simulink model "power_sys_sim"  (R2023b)
settings: Solver=VariableStepAuto  StartTime=0.0  StopTime=0.1  FixedStep=0.00001  RelTol=1e-3
libraries: spsThyristorLib x5, spsVoltageMeasurementLib x5, spsCurrentMeasurementLib x4, spsDiodeLib x4, spsSeriesRLCBranchLib x4, spsACVoltageSourceLib x3, spsMeanLib x2, sps_lib x1
settings Model: Creator=yuanluochen  LastModifiedBy=yuanluochen

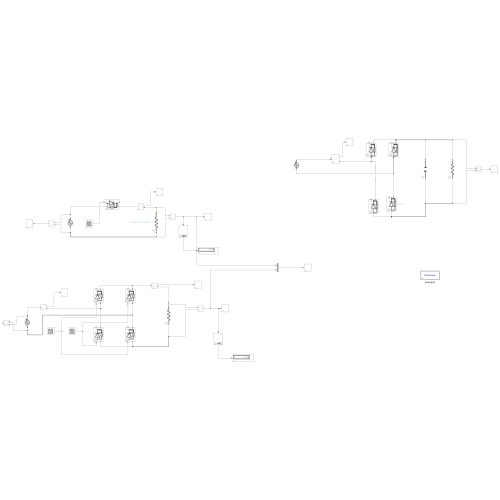
[thumbnail: Simulink's stored preview of the top-level diagram]
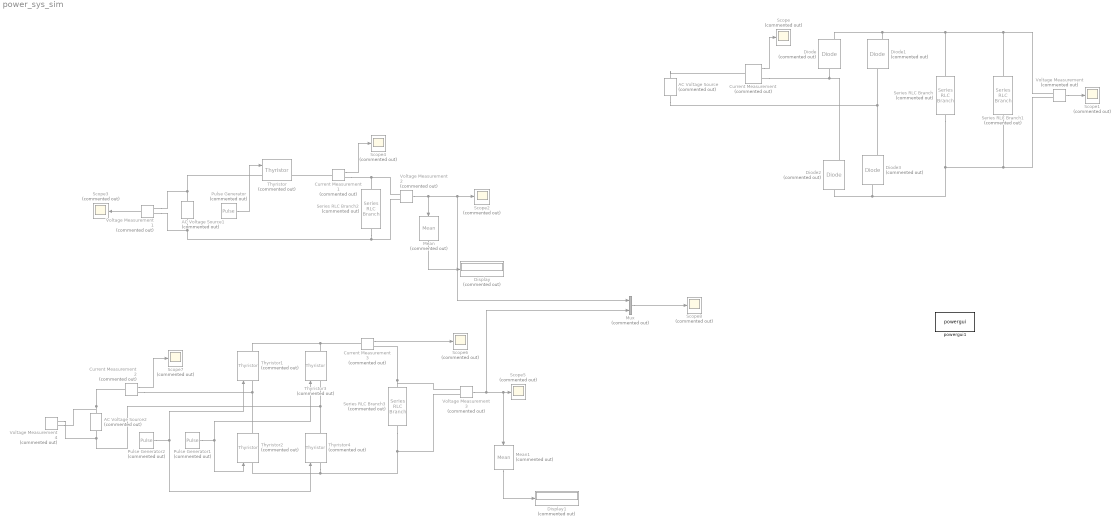
== system power_sys_sim ==
  AC Voltage Source : spsACVoltageSourceLib/AC Voltage Source  Commented=on  Amplitude=220*sqrt(2)  Phase=0  Frequency=50  SampleTime=0  Measurements=None  BusType=swing  Pref=10e3  Qref=0  Qmin=-inf  Qmax=+inf
  AC Voltage Source1 : spsACVoltageSourceLib/AC Voltage Source  Commented=on  Amplitude=220*sqrt(2)  Phase=0  Frequency=50  SampleTime=0  Measurements=None  BusType=swing  Pref=10e3  Qref=0  Qmin=-inf  Qmax=+inf
  AC Voltage Source2 : spsACVoltageSourceLib/AC Voltage Source  Commented=on  Amplitude=220*sqrt(2)  Phase=0  Frequency=50  SampleTime=0  Measurements=None  BusType=swing  Pref=10e3  Qref=0  Qmin=-inf  Qmax=+inf
  Current Measurement{,1..3} (4 alike) : spsCurrentMeasurementLib/Current Measurement  Commented=on  PhasorSimulation=off  OutputType=Complex  PSBequivalent=0
  Diode{,1..3} (4 alike) : spsDiodeLib/Diode  Commented=on  Ron=0.001  Lon=0  Vf=0.8  IC=0  UseSnubber=0  Rs=500  Cs=250e-9  Measurements=on
  Display : Display  Commented=on
  Display1 : Display  Commented=on
  Mean : spsMeanLib/Mean  Commented=on  Freq=50  Vinit=0  Ts=0
  Mean1 : spsMeanLib/Mean  Commented=on  Freq=50  Vinit=0  Ts=0
  Mux : Mux  Commented=on  Inputs=2
  Pulse Generator : DiscretePulseGenerator  Commented=on  PulseType=Time based  Amplitude=3  Period=0.02  PulseWidth=10  PhaseDelay=60/360*0.02
  Pulse Generator1 : DiscretePulseGenerator  Commented=on  PulseType=Time based  Amplitude=3  Period=0.02  PulseWidth=10  PhaseDelay=60/360*0.02+0.01
  Pulse Generator2 : DiscretePulseGenerator  Commented=on  PulseType=Time based  Amplitude=3  Period=0.02  PulseWidth=10  PhaseDelay=60/360*0.02
  Scope{,1..8} (9 alike) : Scope  Commented=on
  Series RLC Branch : spsSeriesRLCBranchLib/Series RLC Branch  Commented=on  LConnTagsString=__new0  RConnTagsString=__new0  BranchType=C  Resistance=1  Inductance=1e-3  SetiL0=off  InitialCurrent=0  Capacitance=0.001  Setx0=off  InitialVoltage=0  Measurements=None
  Series RLC Branch1 : spsSeriesRLCBranchLib/Series RLC Branch  Commented=on  LConnTagsString=__new0  RConnTagsString=__new0  BranchType=R  Resistance=20  Inductance=1e-3  SetiL0=off  InitialCurrent=0  Capacitance=1e-6  Setx0=off  InitialVoltage=0  Measurements=None
  Series RLC Branch2 : spsSeriesRLCBranchLib/Series RLC Branch  Commented=on  LConnTagsString=__new0  RConnTagsString=__new0  BranchType=R  Resistance=20  Inductance=1e-3  SetiL0=off  InitialCurrent=0  Capacitance=1e-6  Setx0=off  InitialVoltage=0  Measurements=None
  Series RLC Branch3 : spsSeriesRLCBranchLib/Series RLC Branch  Commented=on  LConnTagsString=__new0  RConnTagsString=__new0  BranchType=R  Resistance=20  Inductance=1e-3  SetiL0=off  InitialCurrent=0  Capacitance=1e-6  Setx0=off  InitialVoltage=0  Measurements=None
  Thyristor{,1..4} (5 alike) : spsThyristorLib/Thyristor  Commented=on  Ron=0.001  Lon=0  Vf=0.8  IC=0  Rs=500  Cs=250e-9  Measurements=on
  Voltage Measurement{,1..4} (5 alike) : spsVoltageMeasurementLib/Voltage Measurement  Commented=on  PhasorSimulation=off  OutputType=Complex  PSBequivalent=0
  powergui1 : sps_lib/powergui  Priority=1  SimulationMode=Continuous  SampleTime=50e-6  frequency=60  Iterations=50  frequencyindice=50  Pbase=100e6  ErrMax=1e-4  UnitsV=kV  UnitsW=MW  buscounter=0  FunctionMessages=off  echomessages=off  EnableUseOfTLC=off  CurrentSourceSwitches=off  DisableSnubberDevices=off  DisableRonSwitches=off  DisableVfSwitches=off  DisplayEquations=off  AutomaticDiscreteSolvers=off  SolverType=Tustin/Backward Euler (TBE)  Interpol=off  ExternalGateDelay=off  methode=off  Ts=100  x0status=blocks  SPID=on  SwTol=0  HookPort=off  NonlinearTolerance=1e-4  nMaxIteration=100  ContinueOnMaxIteration=off  RestoreLinks=warning  ResistiveCurrentMeasurement=off  Frange=[0:2:500]  Ylog=off  Xlog=on  ShowGrid=off  save=off  variable=ZData  structure=0  ZoomFFT=off  StartTime=0.0  cycles=1  DisplayStyle=1  fundamental=60  FreqAxis=off  MaxFrequency=1000  frequencyindicesteady=1  RmsSteady=1  display=off
  wires:
  Current Measurement/1 -> Scope/1
  Voltage Measurement/1 -> Scope1/1
  Pulse Generator/1 -> Thyristor/1
  Voltage Measurement2/1 -> Mux/1, Scope2/1, Mean/1
  Voltage Measurement1/1 -> Scope3/1
  Mean/1 -> Display/1
  Current Measurement1/1 -> Scope4/1
  Pulse Generator1/1 -> Thyristor3/1, Thyristor2/1
  Pulse Generator2/1 -> Thyristor1/1, Thyristor4/1
  Voltage Measurement3/1 -> Mux/2, Mean1/1, Scope5/1
  Mean1/1 -> Display1/1
  Current Measurement3/1 -> Scope6/1
  Current Measurement2/1 -> Scope7/1
  Mux/1 -> Scope8/1
  connections:
  Diode/LConn1 -- Current Measurement/RConn1 -- Diode2/RConn1
  Diode2/LConn1 -- Series RLC Branch1/RConn1 -- Voltage Measurement/LConn2 -- Series RLC Branch/RConn1 -- Diode3/LConn1
  Diode3/RConn1 -- AC Voltage Source/LConn1 -- Diode1/LConn1
  Diode/RConn1 -- Series RLC Branch1/LConn1 -- Voltage Measurement/LConn1 -- Series RLC Branch/LConn1 -- Diode1/RConn1
  AC Voltage Source/RConn1 -- Current Measurement/LConn1
  AC Voltage Source1/RConn1 -- Thyristor/LConn1 -- Voltage Measurement1/LConn2
  Current Measurement1/LConn1 -- Thyristor/RConn1
  Current Measurement1/RConn1 -- Voltage Measurement2/LConn1 -- Series RLC Branch2/LConn1
  Series RLC Branch2/RConn1 -- Voltage Measurement1/LConn1 -- AC Voltage Source1/LConn1 -- Voltage Measurement2/LConn2
  Thyristor2/RConn1 -- Thyristor1/LConn1 -- Current Measurement2/RConn1
  Thyristor4/RConn1 -- Voltage Measurement4/LConn2 -- AC Voltage Source2/LConn1 -- Thyristor3/LConn1
  Thyristor4/LConn1 -- Voltage Measurement3/LConn2 -- Series RLC Branch3/RConn1 -- Thyristor2/LConn1
  Thyristor3/RConn1 -- Current Measurement3/LConn1 -- Thyristor1/RConn1
  AC Voltage Source2/RConn1 -- Current Measurement2/LConn1 -- Voltage Measurement4/LConn1
  Series RLC Branch3/LConn1 -- Current Measurement3/RConn1 -- Voltage Measurement3/LConn1
